simulink model "Rover"  (R2018b)
settings: Solver=VariableStepAuto  StartTime=0.0  StopTime=100000  FixedStep=1/800  RelTol=1e-3
libraries: AP_Conector x2, robotmobilelib x1

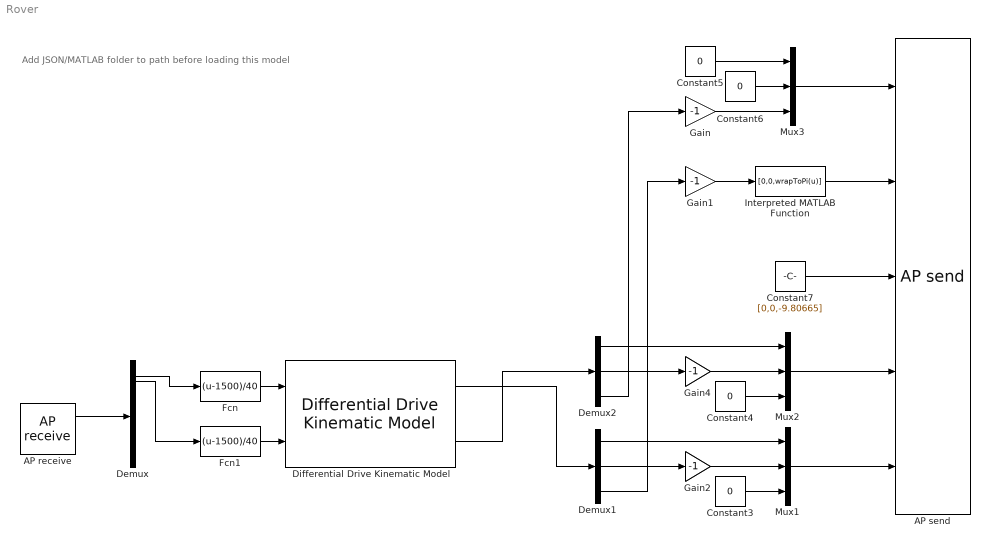
== system Rover ==
  note: Add JSON/MATLAB folder to path before loading this model
  AP receive : AP_Conector/AP receive  SystemSampleTime=-1  Latency=0  AutoFrameSizeCalculation=off
  AP send : AP_Conector/AP send  SystemSampleTime=-1  Latency=0  AutoFrameSizeCalculation=off
  Constant{3..6} (4 alike) : Constant  Value=0
  Constant7 : Constant  Value=[0,0,-9.80665]
  Demux : Demux  Outputs=16
  Demux1 : Demux  Outputs=3
  Demux2 : Demux  Outputs=3
  Differential Drive Kinematic Model : robotmobilelib/Differential Drive Kinematic Model  VehicleInputs=Wheel Speeds  WheelRadius=0.16  WheelSpeedRange=[-100 100]  TrackWidth=0.2  InitialState=[0; 0; 0]  SimulateUsing=Interpreted execution
  Fcn : Fcn  Expr=(u-1500)/40
  Fcn1 : Fcn  Expr=(u-1500)/40
  Gain{,1..2,4} (4 alike) : Gain  Gain=-1
  Interpreted MATLAB Function : MATLABFcn  MATLABFcn=[0,0,wrapToPi(u)]
  Mux1 : Mux  Inputs=3
  Mux2 : Mux  Inputs=3
  Mux3 : Mux  Inputs=3
  wires:
  Fcn/1 -> Differential Drive Kinematic Model/1
  Demux1/3 -> Gain1/1
  Interpreted MATLAB Function/1 -> AP send/2
  Mux1/1 -> AP send/5
  Demux1/2 -> Gain2/1
  Constant3/1 -> Mux1/3
  Constant4/1 -> Mux2/3
  Demux2/2 -> Gain4/1
  Demux2/1 -> Mux2/1
  Mux3/1 -> AP send/1
  Constant6/1 -> Mux3/2
  Constant5/1 -> Mux3/1
  Demux2/3 -> Gain/1
  Mux2/1 -> AP send/4
  Gain/1 -> Mux3/3
  Gain1/1 -> Interpreted MATLAB Function/1
  Demux1/1 -> Mux1/1
  Gain2/1 -> Mux1/2
  Gain4/1 -> Mux2/2
  Demux/2 -> Fcn1/1
  Demux/1 -> Fcn/1
  AP receive/1 -> Demux/1
  Differential Drive Kinematic Model/2 -> Demux2/1
  Differential Drive Kinematic Model/1 -> Demux1/1
  Fcn1/1 -> Differential Drive Kinematic Model/2
  Constant7/1 -> AP send/3
